simulink model "MIL_PIL_Simulation_2022"  (R2020b)
settings: Solver=FixedStepAuto  StartTime=0.0  StopTime=3  FixedStep=0.0001  RelTol=1e-3
values from neighbouring files (symbols this model uses):
  F = 1/(C_aug*inv(eye(5)-phi_aug-Gamma_aug*K)*Gamma_aug)    [Suspension_controller_LQR.m]
  K = -G    [Suspension_controller_LQR.m]
undefined symbols (not defined in the file or in its folder): A_dp, Ad_plant, B_dp, Bd_plant, C_dp, Cd_plant, D_dp, Dd_plant, delay_count, delay_count_dcmotor, F_DCmotor, hc, hp, K_DCmotor, reference, Tp_DC, Ts_DC
settings Model: ExtModeTrigDuration=200  Creator=young  LastModifiedBy=LYD
settings DataIOCC: SaveOutput=off  SaveTime=off  ReturnWorkspaceOutputs=off
settings OptimizationCC: EnhancedBackFolding=on  PassReuseOutputArgsAs=Individual arguments  OptimizeBlockOrder=speed  DifferentSizesBufferReuse=on  OptimizationCustomize=off  EfficientTunableParamExpr=on
settings DebuggingCC: ParameterTunabilityLossMsg=error  ArithmeticOperatorsInVariantConditions=warning
settings HardwareCC: ProdBitPerPointer=32  ProdBitPerSizeT=32  ProdBitPerPtrDiffT=32  ProdLargestAtomicInteger=Integer  ProdLargestAtomicFloat=None  ProdWordSize=32  ProdLongLongMode=on  ProdHWDeviceType=Custom Processor
settings SFSimCC: SimUseLocalCustomCode=off  MATLABDynamicMemAlloc=off  CustomCodeUndefinedFunction=UseInterfaceOnly
settings RTWCC: Description=CompSOC EC Target  SystemTargetFile=CompSOC_ec.tlc  TemplateMakefile=CompSOC_ec.tmf  RTWUseLocalCustomCode=off  IncludeHyperlinkInReport=on  CreateSILPILBlock=PIL  CodeExecutionProfiling=on  CodeProfilingSaveOptions=AllData  CodeProfilingInstrumentation=detailed
settings CodeAppCC: ForceParamTrailComments=on  IgnoreCustomStorageClasses=off  OperatorAnnotations=on  SimulinkDataObjDesc=on  SFDataObjDesc=on  InsertBlockDesc=on
settings STFCustomTargetCC: TargetLibSuffix=.a  TargetLangStandard=C99 (ISO)  MultiwordLength=256  GenerateSampleERTMain=on  ConcurrentExecutionCompliant=off  CombineOutputUpdateFcns=on  ERTCustomFileBanners=on  SupportNonInlinedSFcns=off  RemoveResetFunc=on  MATLABClassNameForMDSCustomization=Simulink.SoftwareTarget.ERTCustomization  CPPClassGenCompliant=off  GRTInterface=off  SystemTargetFile=CompSOC_ec.tlc
settings ERTTargetCC: TargetLangStandard=C99 (ISO)  GenerateSampleERTMain=on  ParMdlRefBuildCompliant=off  CompOptLevelCompliant=off  ConcurrentExecutionCompliant=off  SupportContinuousTime=on  ModelStepFunctionPrototypeControlCompliant=off  CPPClassGenCompliant=off  UseToolchainInfoCompliant=off  ExtMode=on  ExtModeStaticAlloc=on  ExtModeStaticAllocSize=30000  ExtModeMexArgs='10.42.0.229' 1 9878  ERTCustomFileTemplate=CompSOC_ec_file_process.tlc

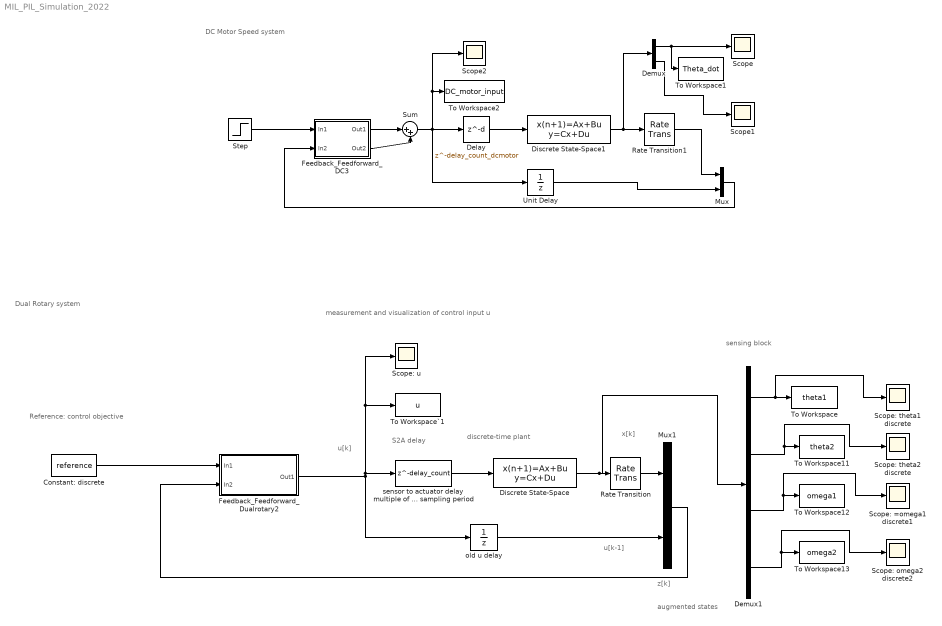
== system MIL_PIL_Simulation_2022 ==
  note: discrete-time plant
  note: sensing block
  note: u[k]
  note: x[k]
  note: measurement and visualization
      | of control input u
  note: augmented states
  note: Reference:
      | control objective
  note: z[k]
  note: u[k-1]
  note: S2A delay
  note: DC Motor Speed system
  note: Dual Rotary system
  Constant: discrete : Constant  Value=reference  OutDataTypeStr=single  SampleTime=hc
  Delay : Delay  DelayLength=delay_count_dcmotor  SampleTime=Tp_DC
  Demux : Demux  Outputs=2
  Demux1 : Demux
  Discrete State-Space : DiscreteStateSpace  A=Ad_plant  B=Bd_plant  C=Cd_plant  D=Dd_plant  SampleTime=hp
  Discrete State-Space1 : DiscreteStateSpace  A=A_dp  B=B_dp  C=C_dp  D=D_dp  SampleTime=Tp_DC
  Feedback_Feedforward_DC3 : Subsystem
  Feedback_Feedforward_Dualrotary2 : Subsystem
  Mux : Mux  Inputs=2
  Mux1 : Mux  Inputs=2
  Rate Transition : RateTransition  Deterministic=off  OutPortSampleTime=hc
  Rate Transition1 : RateTransition  OutPortSampleTime=Ts_DC
  Scope : Scope
  Scope1 : Scope
  Scope2 : Scope
  Scope: =omega1 discrete1 : Scope
  Scope: omega2 discrete2 : Scope
  Scope: theta1 discrete : Scope
  Scope: theta2 discrete : Scope
  Scope: u : Scope
  Step : Step  Time=0  SampleTime=Ts_DC
  Sum : Sum  Inputs=|++
  To Workspace : ToWorkspace  VariableName=theta1  SaveFormat=Timeseries  SampleTime=hc
  To Workspace1 : ToWorkspace  VariableName=Theta_dot  SaveFormat=Timeseries  SampleTime=Tp_DC
  To Workspace11 : ToWorkspace  VariableName=theta2  SaveFormat=Timeseries  SampleTime=hc
  To Workspace12 : ToWorkspace  VariableName=omega1  SaveFormat=Timeseries  SampleTime=hc
  To Workspace13 : ToWorkspace  VariableName=omega2  SaveFormat=Timeseries  SampleTime=hc
  To Workspace2 : ToWorkspace  VariableName=DC_motor_input  SaveFormat=Timeseries  SampleTime=Ts_DC
  To Workspace`1 : ToWorkspace  VariableName=u  SaveFormat=Timeseries  SampleTime=hc
  Unit Delay : UnitDelay  SampleTime=Ts_DC  HasFrameUpgradeWarning=on
  old u delay : UnitDelay  SampleTime=hc  HasFrameUpgradeWarning=on
  sensor to actuator delay multiple of plant sampling period : Delay  DelayLength=delay_count  SampleTime=hp
  wires:
  Unit Delay/1 -> Mux/2
  Discrete State-Space/1 -> Rate Transition/1, Demux1/1
  Delay/1 -> Discrete State-Space1/1
  Rate Transition1/1 -> Mux/1
  Sum/1 -> Unit Delay/1, To Workspace2/1, Scope2/1, Delay/1
  Demux1/3 -> Scope: =omega1 discrete1/1, To Workspace12/1
  Rate Transition/1 -> Mux1/1
  old u delay/1 -> Mux1/2
  Demux1/2 -> Scope: theta2 discrete/1, To Workspace11/1
  sensor to actuator delay multiple of plant sampling period/1 -> Discrete State-Space/1
  Demux1/1 -> Scope: theta1 discrete/1, To Workspace/1
  Discrete State-Space1/1 -> Demux/1, Rate Transition1/1
  Demux1/4 -> Scope: omega2 discrete2/1, To Workspace13/1
  Demux/1 -> To Workspace1/1, Scope/1
  Demux/2 -> Scope1/1
  Step/1 -> Feedback_Feedforward_DC3/1(In1)
  Mux/1 -> Feedback_Feedforward_DC3/2(In2)
  Feedback_Feedforward_DC3/1(Out1) -> Sum/1
  Feedback_Feedforward_DC3/2(Out2) -> Sum/2
  Feedback_Feedforward_Dualrotary2/1(Out1) -> sensor to actuator delay multiple of plant sampling period/1, Scope: u/1, To Workspace`1/1, old u delay/1
  Mux1/1 -> Feedback_Feedforward_Dualrotary2/2(In2)
  Constant: discrete/1 -> Feedback_Feedforward_Dualrotary2/1(In1)

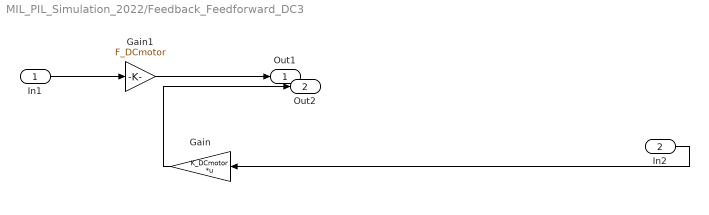
== system MIL_PIL_Simulation_2022/Feedback_Feedforward_DC3 ==
  In1 : Inport
  In2 : Inport  Port=2
  Gain : Gain  Gain=K_DCmotor  Multiplication=Matrix(K*u) (u vector)
  Gain1 : Gain  Gain=F_DCmotor
  Out1 : Outport  VectorParamsAs1DForOutWhenUnconnected=off
  Out2 : Outport  Port=2  VectorParamsAs1DForOutWhenUnconnected=off
  wires:
  Gain1/1 -> Out1/1
  In2/1 -> Gain/1
  In1/1 -> Gain1/1
  Gain/1 -> Out2/1

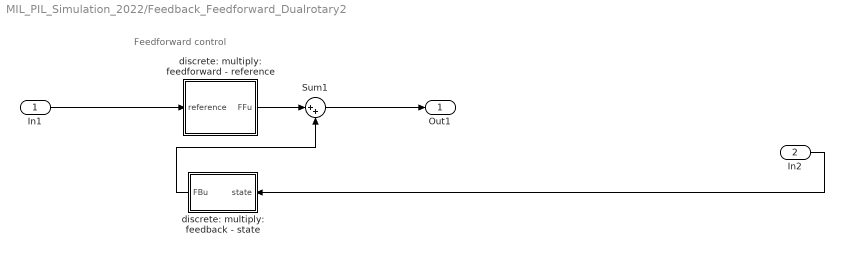
== system MIL_PIL_Simulation_2022/Feedback_Feedforward_Dualrotary2 ==
  note: Feedforward control
  In1 : Inport
  In2 : Inport  Port=2
  Sum1 : Sum  Inputs=|++
  discrete: multiply: feedback - state : Subsystem
  discrete: multiply: feedforward - reference : Subsystem
  Out1 : Outport  VectorParamsAs1DForOutWhenUnconnected=off
  wires:
  In1/1 -> discrete: multiply: feedforward - reference/1(reference)
  discrete: multiply: feedback - state/1(FBu) -> Sum1/2
  discrete: multiply: feedforward - reference/1(FFu) -> Sum1/1
  Sum1/1 -> Out1/1
  In2/1 -> discrete: multiply: feedback - state/1(state)

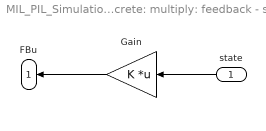
== system MIL_PIL_Simulation_2022/Feedback_Feedforward_Dualrotary2/discrete: multiply: feedback - state ==
  state : Inport  OutDataTypeStr=single  SampleTime=hc
  Gain : Gain  Gain=K  Multiplication=Matrix(K*u) (u vector)  OutDataTypeStr=single
  FBu : Outport  OutDataTypeStr=single  SampleTime=hc  InitialOutput=[0]  VectorParamsAs1DForOutWhenUnconnected=off
  wires:
  state/1 -> Gain/1
  Gain/1 -> FBu/1

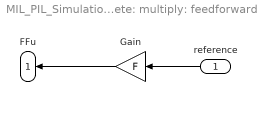
== system MIL_PIL_Simulation_2022/Feedback_Feedforward_Dualrotary2/discrete: multiply: feedforward - reference ==
  reference : Inport  OutDataTypeStr=single  SampleTime=hc
  Gain : Gain  Gain=F  OutDataTypeStr=single
  FFu : Outport  OutDataTypeStr=single  SampleTime=hc  InitialOutput=[0]  VectorParamsAs1DForOutWhenUnconnected=off
  wires:
  reference/1 -> Gain/1
  Gain/1 -> FFu/1
